simulink model "root"  (R2014a)
settings: Solver=FixedStepDiscrete  StartTime=0.0  StopTime=1  RelTol=1e-3
model workspace (MAT data in the model file):
  Fs = 48000
  dtmfFramesize = 256
undefined symbols (not defined in the file): jet
libraries: DSPBAPrim x6, dspsnks4 x2, dspspect3 x1, dspmathops x1, dspswit3 x1
settings Model: Creator=User  LastModifiedBy=User
settings OptimizationCC: BlockReduction=off  ConditionallyExecuteInputs=off  InlineParams=on
settings HardwareCC: ProdHWDeviceType=ASIC/FPGA->ASIC/FPGA  TargetLongLongMode=on  TargetIntDivRoundTo=Zero  TargetEndianess=LittleEndian  TargetHWDeviceType=MATLAB Host  ProdEqTarget=off

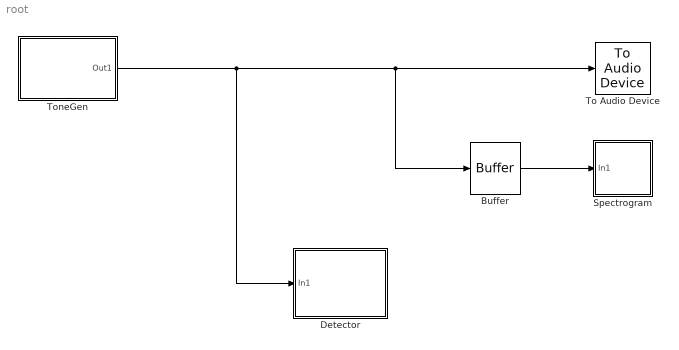
== system root ==
  Buffer : Buffer  N=dtmfFramesize  TreatMby1Signals=One channel
  Detector : Subsystem
  Spectrogram : Subsystem
  To Audio Device : dspsnks4/To Audio Device  deviceName=Default  inheritSampleRate=on  sampleRate=44100  deviceDatatype=Determine from input data type  autoBufferSize=on  bufferSize=4096  queueDuration=1.0  defaultOutputChannelMapping=on  outputChannelMapping=1
  ToneGen : Subsystem
  wires:
  ToneGen/1(Out1) -> Detector/1(In1), Buffer/1, To Audio Device/1
  Buffer/1 -> Spectrogram/1(In1)

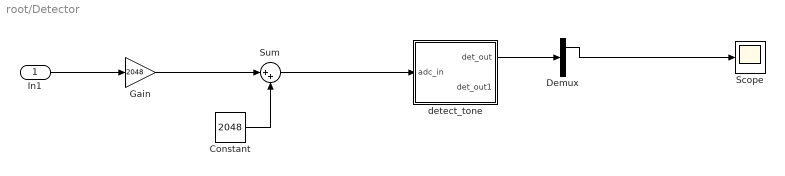
== system root/Detector ==
  In1 : Inport
  Constant : Constant  Value=2048  OutDataTypeStr=fixdt(0,12,0)
  Demux : Demux  Outputs=3
  Gain : Gain  Gain=2048
  Scope : Scope
      settings: YMin=1  YMax=1  MaxDataPoints=500000
  Sum : Sum  Inputs=|++  OutDataTypeStr=fixdt(0,12,0)
  detect_tone : Subsystem
  wires:
  In1/1 -> Gain/1
  Gain/1 -> Sum/1
  Constant/1 -> Sum/2
  Sum/1 -> detect_tone/1(adc_in)
  detect_tone/1(det_out) -> Demux/1
  Demux/1 -> Scope/1

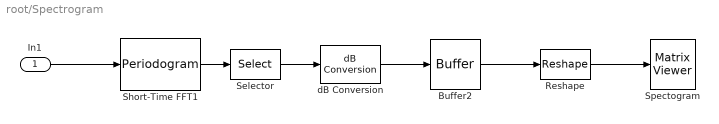
== system root/Spectrogram ==
  In1 : Inport
  Buffer2 : Buffer  N=48*64  V=46*64  ic=-70  TreatMby1Signals=One channel
  Reshape : Reshape  OutputDimensionality=Customize  OutputDimensions=[64 48]
  Selector : Selector  InputPortWidth=dtmfFramesize/2  Indices=1:(dtmfFramesize/4)
  Short-Time FFT1 : dspspect3/Periodogram  measurement=Power spectral density  wintype=Hamming  Rs=50  beta=5  winsamp=Periodic  FFTImplementation=Auto  inheritFFT=off  fftsize=128  navg=2  inheritTs=on  Ts=1
  Spectogram : dspsnks4/Matrix Viewer  ImageParams=on  CMapStr=jet(256)  AxisColorbar=off  AxisParams=on  AxisOrigin=Lower left corner  XLabel=Time Index  YLabel=Frequency Index  ZLabel=dB Magnitude  FigPos=[214 452 283 114]  AxisZoom=on
      settings: YMin=-150  YMax=-65
  dB Conversion : dspmathops/dB Conversion  dBtype=dB  intype=Amplitude  R=1  fuzz=on
  wires:
  Short-Time FFT1/1 -> Selector/1
  Selector/1 -> dB Conversion/1
  Buffer2/1 -> Reshape/1
  In1/1 -> Short-Time FFT1/1
  Reshape/1 -> Spectogram/1
  dB Conversion/1 -> Buffer2/1

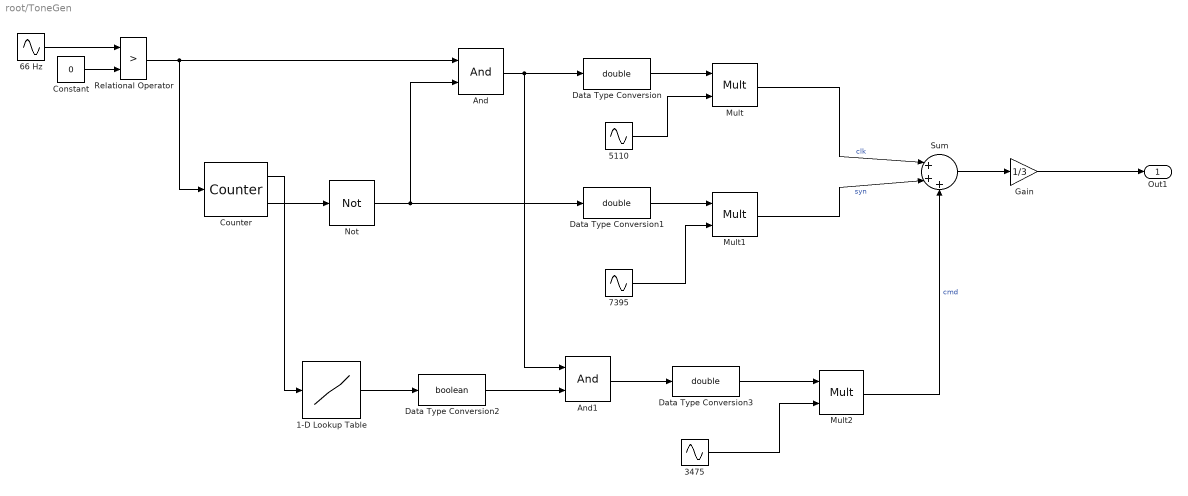
== system root/ToneGen ==
  1-D Lookup Table : Lookup_n-D  NumberOfTableDimensions=1  BreakpointsForDimension1=[0:15]  Table=[0 1 0 1 1 0 1 0 0 1 0 1 0 0 1 1]  InternalRulePriority=Speed  RndMeth=Simplest  InputSameDT=on
  3475 : Sin  Frequency=3475*2*pi  SampleTime=1/Fs
  5110 : Sin  Frequency=5110*2*pi  SampleTime=1/Fs
  66 Hz : Sin  Frequency=66*2*pi  SampleTime=1/Fs
  7395 : Sin  Frequency=7395*2*pi  SampleTime=1/Fs
  And : DSPBAPrim/And  primtype=and  nInputs=2  nOutputs=1  omode=Inherit via internal rule  otype=sfix(16)  scale=2^-15  rndmethod=Unbiased  factor=1  satmethod=Symmetric  shift_vec=[0 1 2 -1]  value=0  inPortNames=[' '; ' '; ' '; ' '; ' '; ' '; ' '; ' '; ' '; ' '; ' '; ' '; ' '; ' '; ' '; ' '; ]  outPortNames=[' ']  dspbaimage=dspba_prim.jpg  text=fprintf('&');  style=Optimised  visibilities=8+2  version=20090407
  And1 : DSPBAPrim/And  primtype=and  nInputs=2  nOutputs=1  omode=Inherit via internal rule  otype=sfix(16)  scale=2^-15  rndmethod=Unbiased  factor=1  satmethod=Symmetric  shift_vec=[0 1 2 -1]  value=0  inPortNames=[' '; ' '; ' '; ' '; ' '; ' '; ' '; ' '; ' '; ' '; ' '; ' '; ' '; ' '; ' '; ' '; ]  outPortNames=[' ']  dspbaimage=dspba_prim.jpg  text=fprintf('&');  style=Optimised  visibilities=8+2  version=20090407
  Constant : Constant  Value=0
  Counter : dspswit3/Counter  Direction=Up  CountEvent=Rising edge  CounterSize=User defined  MaxCount=15  InitialCount=0  Output=Count and Hit  HitValue=0  ResetInput=off  SamplesPerFrame=1  Ts=1  CntDtype=double  HitDtype=Logical
  Data Type Conversion : DataTypeConversion  OutDataTypeStr=double
  Data Type Conversion1 : DataTypeConversion  OutDataTypeStr=double
  Data Type Conversion2 : DataTypeConversion  OutDataTypeStr=boolean
  Data Type Conversion3 : DataTypeConversion  OutDataTypeStr=double
  Gain : Gain  Gain=1/3
  Mult : DSPBAPrim/Mult  primtype=mult  nInputs=2  nOutputs=1  omode=Inherit via internal rule  otype=sfix(16)  scale=2^-15  rndmethod=Unbiased  factor=1  satmethod=Symmetric  shift_vec=[0 1 2 -1]  value=0  inPortNames=[' '; ' ';]  outPortNames=[' ']  dspbaimage=dspba_prim.jpg  text=fprintf('X');  style=Optimised  visibilities=8  version=20090407
  Mult1 : DSPBAPrim/Mult  primtype=mult  nInputs=2  nOutputs=1  omode=Inherit via internal rule  otype=sfix(16)  scale=2^-15  rndmethod=Unbiased  factor=1  satmethod=Symmetric  shift_vec=[0 1 2 -1]  value=0  inPortNames=[' '; ' ';]  outPortNames=[' ']  dspbaimage=dspba_prim.jpg  text=fprintf('X');  style=Optimised  visibilities=8  version=20090407
  Mult2 : DSPBAPrim/Mult  primtype=mult  nInputs=2  nOutputs=1  omode=Inherit via internal rule  otype=sfix(16)  scale=2^-15  rndmethod=Unbiased  factor=1  satmethod=Symmetric  shift_vec=[0 1 2 -1]  value=0  inPortNames=[' '; ' ';]  outPortNames=[' ']  dspbaimage=dspba_prim.jpg  text=fprintf('X');  style=Optimised  visibilities=8  version=20090407
  Not : DSPBAPrim/Not  primtype=not  nInputs=1  nOutputs=1  omode=Inherit via internal rule  otype=sfix(16)  scale=2^-15  rndmethod=Unbiased  factor=1  satmethod=Symmetric  shift_vec=[0 1 2 -1]  value=0  inPortNames=[' '; ' ';]  outPortNames=[' ']  dspbaimage=dspba_prim.jpg  text=fprintf('~');  style=Optimised  visibilities=8  version=20090407
  Relational Operator : RelationalOperator  Operator=>  OutDataTypeStr=boolean
  Sum : Sum  Inputs=|+++
  Out1 : Outport
  wires:
  66 Hz/1 -> Relational Operator/1
  Constant/1 -> Relational Operator/2
  Relational Operator/1 -> And/1, Counter/1
  Data Type Conversion/1 -> Mult/1
  5110/1 -> Mult/2
  Counter/2 -> Not/1
  Not/1 -> And/2, Data Type Conversion1/1
  7395/1 -> Mult1/2
  Sum/1 -> Gain/1
  Mult/1 -> Sum/1  "clk"
  Mult1/1 -> Sum/2  "syn"
  Mult2/1 -> Sum/3  "cmd"
  Data Type Conversion1/1 -> Mult1/1
  3475/1 -> Mult2/2
  Counter/1 -> 1-D Lookup Table/1
  1-D Lookup Table/1 -> Data Type Conversion2/1
  And/1 -> And1/1, Data Type Conversion/1
  And1/1 -> Data Type Conversion3/1
  Data Type Conversion2/1 -> And1/2
  Data Type Conversion3/1 -> Mult2/1
  Gain/1 -> Out1/1

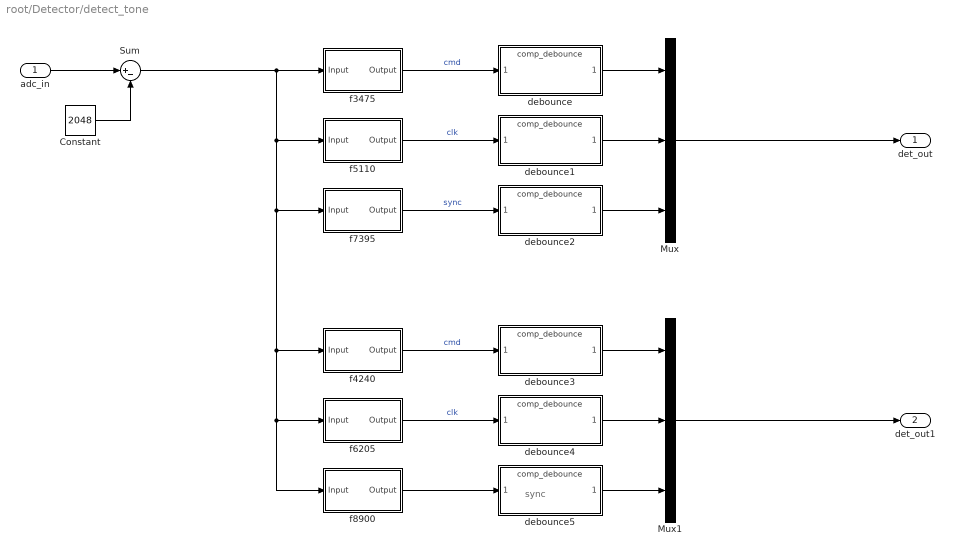
== system root/Detector/detect_tone ==
  note: sync
  adc_in : Inport  OutDataTypeStr=fixdt(0,12,0)
  Constant : Constant  Value=2048  OutDataTypeStr=fixdt(1,16,0)
  Mux : Mux  Inputs=3
  Mux1 : Mux  Inputs=3
  Sum : Sum  Inputs=|+-  AccumDataTypeStr=fixdt(1,16,0)
  debounce{,1..5} (6 alike) : ModelReference  ModelNameDialog=comp_debounce.slx  SimulationMode=Normal  ModelReferenceVersion=1.4  CopyOfModelName=comp_debounce.slx  DefaultDataLogging=on
  f3475 : Subsystem  Tag=FilterWizardSubSystem
      settings: ErrorFcn=dspFilterRealizedInBasicElemsAlgLoopErrFcnCallback
  f4240 : Subsystem  Tag=FilterWizardSubSystem
      settings: ErrorFcn=dspFilterRealizedInBasicElemsAlgLoopErrFcnCallback
  f5110 : Subsystem  Tag=FilterWizardSubSystem
      settings: ErrorFcn=dspFilterRealizedInBasicElemsAlgLoopErrFcnCallback
  f6205 : Subsystem  Tag=FilterWizardSubSystem
      settings: ErrorFcn=dspFilterRealizedInBasicElemsAlgLoopErrFcnCallback
  f7395 : Subsystem  Tag=FilterWizardSubSystem
      settings: ErrorFcn=dspFilterRealizedInBasicElemsAlgLoopErrFcnCallback
  f8900 : Subsystem  Tag=FilterWizardSubSystem
      settings: ErrorFcn=dspFilterRealizedInBasicElemsAlgLoopErrFcnCallback
  det_out : Outport
  det_out1 : Outport  Port=2
  wires:
  adc_in/1 -> Sum/1
  Constant/1 -> Sum/2
  Sum/1 -> f6205/1(Input), f8900/1(Input), f4240/1(Input), f7395/1(Input), f5110/1(Input), f3475/1(Input)
  f3475/1(Output) -> debounce/1  "cmd"
  f5110/1(Output) -> debounce1/1  "clk"
  f7395/1(Output) -> debounce2/1  "sync"
  Mux/1 -> det_out/1
  Mux1/1 -> det_out1/1
  f4240/1(Output) -> debounce3/1  "cmd"
  f6205/1(Output) -> debounce4/1  "clk"
  f8900/1(Output) -> debounce5/1
  debounce/1 -> Mux/1
  debounce1/1 -> Mux/2
  debounce2/1 -> Mux/3
  debounce3/1 -> Mux1/1
  debounce4/1 -> Mux1/2
  debounce5/1 -> Mux1/3

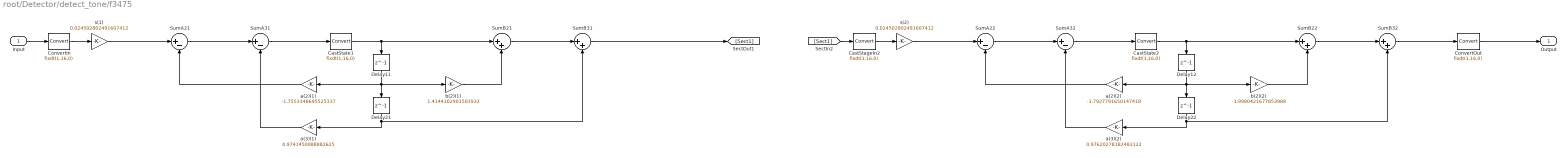
== system root/Detector/detect_tone/f3475 ==
  Input : Inport
  CastStageIn2 : DataTypeConversion  OutDataTypeStr=fixdt(1,16,0)  RndMeth=Convergent  SaturateOnIntegerOverflow=on
  CastState1 : DataTypeConversion  OutDataTypeStr=fixdt(1,16,0)  RndMeth=Convergent  SaturateOnIntegerOverflow=on
  CastState2 : DataTypeConversion  OutDataTypeStr=fixdt(1,16,0)  RndMeth=Convergent  SaturateOnIntegerOverflow=on
  ConvertIn : DataTypeConversion  OutDataTypeStr=fixdt(1,16,0)  RndMeth=Nearest  SaturateOnIntegerOverflow=on
  ConvertOut : DataTypeConversion  OutDataTypeStr=fixdt(1,16,0)  RndMeth=Convergent  SaturateOnIntegerOverflow=on
  Delay{11..12,21..22} (4 alike) : Delay  DelayLength=1  InitialCondition=0
  SumA{21..22,31..32} (4 alike) : Sum  Inputs=|+-  AccumDataTypeStr=fixdt(1,34,14)  OutDataTypeStr=fixdt(1,34,14)  RndMeth=Convergent  SaturateOnIntegerOverflow=on
  SumB{21..22,31..32} (4 alike) : Sum  Inputs=|++  AccumDataTypeStr=fixdt(1,34,14)  OutDataTypeStr=fixdt(1,34,14)  RndMeth=Convergent  SaturateOnIntegerOverflow=on
  a(2)(1) : Gain  Gain=-1.7553348695525337  ParamDataTypeStr=fixdt(1,16,14)  OutDataTypeStr=fixdt(1,32,14)  RndMeth=Convergent  SaturateOnIntegerOverflow=on
  a(2)(2) : Gain  Gain=-1.7927791650147418  ParamDataTypeStr=fixdt(1,16,14)  OutDataTypeStr=fixdt(1,32,14)  RndMeth=Convergent  SaturateOnIntegerOverflow=on
  a(3)(1) : Gain  Gain=0.9741450088882625  ParamDataTypeStr=fixdt(1,16,14)  OutDataTypeStr=fixdt(1,32,14)  RndMeth=Convergent  SaturateOnIntegerOverflow=on
  a(3)(2) : Gain  Gain=0.97620278182483122  ParamDataTypeStr=fixdt(1,16,14)  OutDataTypeStr=fixdt(1,32,14)  RndMeth=Convergent  SaturateOnIntegerOverflow=on
  b(2)(1) : Gain  Gain=1.4144102901503932  ParamDataTypeStr=fixdt(1,16,14)  OutDataTypeStr=fixdt(1,32,14)  RndMeth=Convergent  SaturateOnIntegerOverflow=on
  b(2)(2) : Gain  Gain=-1.9980421677853988  ParamDataTypeStr=fixdt(1,16,14)  OutDataTypeStr=fixdt(1,32,14)  RndMeth=Convergent  SaturateOnIntegerOverflow=on
  s(1) : Gain  Gain=0.024502802491607412  ParamDataTypeStr=fixdt(1,16,20)  OutDataTypeStr=fixdt(1,16,0)  RndMeth=Convergent  SaturateOnIntegerOverflow=on
  s(2) : Gain  Gain=0.024502802491607412  ParamDataTypeStr=fixdt(1,16,20)  OutDataTypeStr=fixdt(1,16,0)  RndMeth=Convergent  SaturateOnIntegerOverflow=on
  Output : Outport
  wires:
  Input/1 -> ConvertIn/1
  s(1)/1 -> SumA21/1
  SumA21/1 -> SumA31/1
  SumA31/1 -> CastState1/1
  CastState1/1 -> SumB21/1, Delay11/1
  SumB21/1 -> SumB31/1
  SumB31/1 -> [Sect1]
  a(2)(1)/1 -> SumA21/2
  Delay11/1 -> a(2)(1)/1, b(2)(1)/1, Delay21/1
  b(2)(1)/1 -> SumB21/2
  a(3)(1)/1 -> SumA31/2
  Delay21/1 -> a(3)(1)/1, SumB31/2
  ConvertIn/1 -> s(1)/1
  [Sect1] -> CastStageIn2/1
  s(2)/1 -> SumA22/1
  SumA22/1 -> SumA32/1
  SumA32/1 -> CastState2/1
  CastState2/1 -> SumB22/1, Delay12/1
  SumB22/1 -> SumB32/1
  SumB32/1 -> ConvertOut/1
  a(2)(2)/1 -> SumA22/2
  Delay12/1 -> a(2)(2)/1, b(2)(2)/1, Delay22/1
  b(2)(2)/1 -> SumB22/2
  a(3)(2)/1 -> SumA32/2
  Delay22/1 -> a(3)(2)/1, SumB32/2
  ConvertOut/1 -> Output/1
  CastStageIn2/1 -> s(2)/1

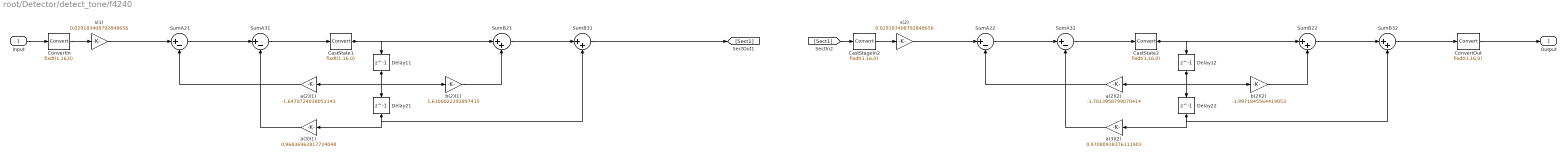
== system root/Detector/detect_tone/f4240 ==
  Input : Inport
  CastStageIn2 : DataTypeConversion  OutDataTypeStr=fixdt(1,16,0)  RndMeth=Convergent  SaturateOnIntegerOverflow=on
  CastState1 : DataTypeConversion  OutDataTypeStr=fixdt(1,16,0)  RndMeth=Convergent  SaturateOnIntegerOverflow=on
  CastState2 : DataTypeConversion  OutDataTypeStr=fixdt(1,16,0)  RndMeth=Convergent  SaturateOnIntegerOverflow=on
  ConvertIn : DataTypeConversion  OutDataTypeStr=fixdt(1,16,0)  RndMeth=Nearest  SaturateOnIntegerOverflow=on
  ConvertOut : DataTypeConversion  OutDataTypeStr=fixdt(1,16,0)  RndMeth=Convergent  SaturateOnIntegerOverflow=on
  Delay{11..12,21..22} (4 alike) : Delay  DelayLength=1  InitialCondition=0
  SumA{21..22,31..32} (4 alike) : Sum  Inputs=|+-  AccumDataTypeStr=fixdt(1,34,14)  OutDataTypeStr=fixdt(1,34,14)  RndMeth=Convergent  SaturateOnIntegerOverflow=on
  SumB{21..22,31..32} (4 alike) : Sum  Inputs=|++  AccumDataTypeStr=fixdt(1,34,14)  OutDataTypeStr=fixdt(1,34,14)  RndMeth=Convergent  SaturateOnIntegerOverflow=on
  a(2)(1) : Gain  Gain=-1.6470724038051143  ParamDataTypeStr=fixdt(1,16,14)  OutDataTypeStr=fixdt(1,32,14)  RndMeth=Convergent  SaturateOnIntegerOverflow=on
  a(2)(2) : Gain  Gain=-1.7013958799070414  ParamDataTypeStr=fixdt(1,16,14)  OutDataTypeStr=fixdt(1,32,14)  RndMeth=Convergent  SaturateOnIntegerOverflow=on
  a(3)(1) : Gain  Gain=0.96836962817724048  ParamDataTypeStr=fixdt(1,16,14)  OutDataTypeStr=fixdt(1,32,14)  RndMeth=Convergent  SaturateOnIntegerOverflow=on
  a(3)(2) : Gain  Gain=0.97080938376111903  ParamDataTypeStr=fixdt(1,16,14)  OutDataTypeStr=fixdt(1,32,14)  RndMeth=Convergent  SaturateOnIntegerOverflow=on
  b(2)(1) : Gain  Gain=1.6100022392897415  ParamDataTypeStr=fixdt(1,16,14)  OutDataTypeStr=fixdt(1,32,14)  RndMeth=Convergent  SaturateOnIntegerOverflow=on
  b(2)(2) : Gain  Gain=-1.9971845564419053  ParamDataTypeStr=fixdt(1,16,14)  OutDataTypeStr=fixdt(1,32,14)  RndMeth=Convergent  SaturateOnIntegerOverflow=on
  s(1) : Gain  Gain=0.029183408792848656  ParamDataTypeStr=fixdt(1,16,20)  OutDataTypeStr=fixdt(1,16,0)  RndMeth=Convergent  SaturateOnIntegerOverflow=on
  s(2) : Gain  Gain=0.029183408792848656  ParamDataTypeStr=fixdt(1,16,20)  OutDataTypeStr=fixdt(1,16,0)  RndMeth=Convergent  SaturateOnIntegerOverflow=on
  Output : Outport
  wires:
  Input/1 -> ConvertIn/1
  s(1)/1 -> SumA21/1
  SumA21/1 -> SumA31/1
  SumA31/1 -> CastState1/1
  CastState1/1 -> SumB21/1, Delay11/1
  SumB21/1 -> SumB31/1
  SumB31/1 -> [Sect1]
  a(2)(1)/1 -> SumA21/2
  Delay11/1 -> a(2)(1)/1, b(2)(1)/1, Delay21/1
  b(2)(1)/1 -> SumB21/2
  a(3)(1)/1 -> SumA31/2
  Delay21/1 -> a(3)(1)/1, SumB31/2
  ConvertIn/1 -> s(1)/1
  [Sect1] -> CastStageIn2/1
  s(2)/1 -> SumA22/1
  SumA22/1 -> SumA32/1
  SumA32/1 -> CastState2/1
  CastState2/1 -> SumB22/1, Delay12/1
  SumB22/1 -> SumB32/1
  SumB32/1 -> ConvertOut/1
  a(2)(2)/1 -> SumA22/2
  Delay12/1 -> a(2)(2)/1, b(2)(2)/1, Delay22/1
  b(2)(2)/1 -> SumB22/2
  a(3)(2)/1 -> SumA32/2
  Delay22/1 -> a(3)(2)/1, SumB32/2
  ConvertOut/1 -> Output/1
  CastStageIn2/1 -> s(2)/1

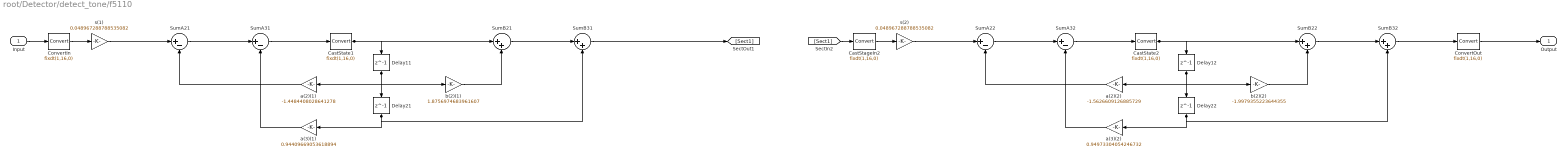
== system root/Detector/detect_tone/f5110 ==
  Input : Inport
  CastStageIn2 : DataTypeConversion  OutDataTypeStr=fixdt(1,16,0)  RndMeth=Convergent  SaturateOnIntegerOverflow=on
  CastState1 : DataTypeConversion  OutDataTypeStr=fixdt(1,16,0)  RndMeth=Convergent  SaturateOnIntegerOverflow=on
  CastState2 : DataTypeConversion  OutDataTypeStr=fixdt(1,16,0)  RndMeth=Convergent  SaturateOnIntegerOverflow=on
  ConvertIn : DataTypeConversion  OutDataTypeStr=fixdt(1,16,0)  RndMeth=Nearest  SaturateOnIntegerOverflow=on
  ConvertOut : DataTypeConversion  OutDataTypeStr=fixdt(1,16,0)  RndMeth=Convergent  SaturateOnIntegerOverflow=on
  Delay{11..12,21..22} (4 alike) : Delay  DelayLength=1  InitialCondition=0
  SumA{21..22,31..32} (4 alike) : Sum  Inputs=|+-  AccumDataTypeStr=fixdt(1,34,14)  OutDataTypeStr=fixdt(1,34,14)  RndMeth=Convergent  SaturateOnIntegerOverflow=on
  SumB{21..22,31..32} (4 alike) : Sum  Inputs=|++  AccumDataTypeStr=fixdt(1,34,14)  OutDataTypeStr=fixdt(1,34,14)  RndMeth=Convergent  SaturateOnIntegerOverflow=on
  a(2)(1) : Gain  Gain=-1.4484408028641278  ParamDataTypeStr=fixdt(1,16,14)  OutDataTypeStr=fixdt(1,32,14)  RndMeth=Convergent  SaturateOnIntegerOverflow=on
  a(2)(2) : Gain  Gain=-1.5626609126885729  ParamDataTypeStr=fixdt(1,16,14)  OutDataTypeStr=fixdt(1,32,14)  RndMeth=Convergent  SaturateOnIntegerOverflow=on
  a(3)(1) : Gain  Gain=0.94409669053618894  ParamDataTypeStr=fixdt(1,16,14)  OutDataTypeStr=fixdt(1,32,14)  RndMeth=Convergent  SaturateOnIntegerOverflow=on
  a(3)(2) : Gain  Gain=0.94973304054246732  ParamDataTypeStr=fixdt(1,16,14)  OutDataTypeStr=fixdt(1,32,14)  RndMeth=Convergent  SaturateOnIntegerOverflow=on
  b(2)(1) : Gain  Gain=1.8756974683961607  ParamDataTypeStr=fixdt(1,16,14)  OutDataTypeStr=fixdt(1,32,14)  RndMeth=Convergent  SaturateOnIntegerOverflow=on
  b(2)(2) : Gain  Gain=-1.9979355223644355  ParamDataTypeStr=fixdt(1,16,14)  OutDataTypeStr=fixdt(1,32,14)  RndMeth=Convergent  SaturateOnIntegerOverflow=on
  s(1) : Gain  Gain=0.048967288788535082  ParamDataTypeStr=fixdt(1,16,19)  OutDataTypeStr=fixdt(1,16,0)  RndMeth=Convergent  SaturateOnIntegerOverflow=on
  s(2) : Gain  Gain=0.048967288788535082  ParamDataTypeStr=fixdt(1,16,19)  OutDataTypeStr=fixdt(1,16,0)  RndMeth=Convergent  SaturateOnIntegerOverflow=on
  Output : Outport
  wires:
  Input/1 -> ConvertIn/1
  s(1)/1 -> SumA21/1
  SumA21/1 -> SumA31/1
  SumA31/1 -> CastState1/1
  CastState1/1 -> SumB21/1, Delay11/1
  SumB21/1 -> SumB31/1
  SumB31/1 -> [Sect1]
  a(2)(1)/1 -> SumA21/2
  Delay11/1 -> a(2)(1)/1, b(2)(1)/1, Delay21/1
  b(2)(1)/1 -> SumB21/2
  a(3)(1)/1 -> SumA31/2
  Delay21/1 -> a(3)(1)/1, SumB31/2
  ConvertIn/1 -> s(1)/1
  [Sect1] -> CastStageIn2/1
  s(2)/1 -> SumA22/1
  SumA22/1 -> SumA32/1
  SumA32/1 -> CastState2/1
  CastState2/1 -> SumB22/1, Delay12/1
  SumB22/1 -> SumB32/1
  SumB32/1 -> ConvertOut/1
  a(2)(2)/1 -> SumA22/2
  Delay12/1 -> a(2)(2)/1, b(2)(2)/1, Delay22/1
  b(2)(2)/1 -> SumB22/2
  a(3)(2)/1 -> SumA32/2
  Delay22/1 -> a(3)(2)/1, SumB32/2
  ConvertOut/1 -> Output/1
  CastStageIn2/1 -> s(2)/1

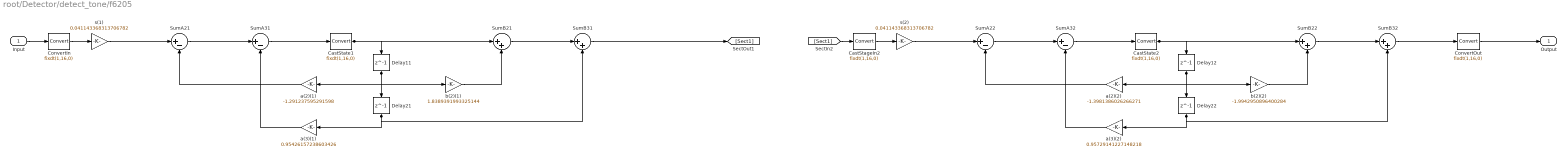
== system root/Detector/detect_tone/f6205 ==
  Input : Inport
  CastStageIn2 : DataTypeConversion  OutDataTypeStr=fixdt(1,16,0)  RndMeth=Convergent  SaturateOnIntegerOverflow=on
  CastState1 : DataTypeConversion  OutDataTypeStr=fixdt(1,16,0)  RndMeth=Convergent  SaturateOnIntegerOverflow=on
  CastState2 : DataTypeConversion  OutDataTypeStr=fixdt(1,16,0)  RndMeth=Convergent  SaturateOnIntegerOverflow=on
  ConvertIn : DataTypeConversion  OutDataTypeStr=fixdt(1,16,0)  RndMeth=Nearest  SaturateOnIntegerOverflow=on
  ConvertOut : DataTypeConversion  OutDataTypeStr=fixdt(1,16,0)  RndMeth=Convergent  SaturateOnIntegerOverflow=on
  Delay{11..12,21..22} (4 alike) : Delay  DelayLength=1  InitialCondition=0
  SumA{21..22,31..32} (4 alike) : Sum  Inputs=|+-  AccumDataTypeStr=fixdt(1,34,14)  OutDataTypeStr=fixdt(1,34,14)  RndMeth=Convergent  SaturateOnIntegerOverflow=on
  SumB{21..22,31..32} (4 alike) : Sum  Inputs=|++  AccumDataTypeStr=fixdt(1,34,14)  OutDataTypeStr=fixdt(1,34,14)  RndMeth=Convergent  SaturateOnIntegerOverflow=on
  a(2)(1) : Gain  Gain=-1.291237595291598  ParamDataTypeStr=fixdt(1,16,14)  OutDataTypeStr=fixdt(1,32,14)  RndMeth=Convergent  SaturateOnIntegerOverflow=on
  a(2)(2) : Gain  Gain=-1.3981386026266271  ParamDataTypeStr=fixdt(1,16,14)  OutDataTypeStr=fixdt(1,32,14)  RndMeth=Convergent  SaturateOnIntegerOverflow=on
  a(3)(1) : Gain  Gain=0.95426157238603426  ParamDataTypeStr=fixdt(1,16,14)  OutDataTypeStr=fixdt(1,32,14)  RndMeth=Convergent  SaturateOnIntegerOverflow=on
  a(3)(2) : Gain  Gain=0.95729141227148218  ParamDataTypeStr=fixdt(1,16,14)  OutDataTypeStr=fixdt(1,32,14)  RndMeth=Convergent  SaturateOnIntegerOverflow=on
  b(2)(1) : Gain  Gain=1.8389391993325144  ParamDataTypeStr=fixdt(1,16,14)  OutDataTypeStr=fixdt(1,32,14)  RndMeth=Convergent  SaturateOnIntegerOverflow=on
  b(2)(2) : Gain  Gain=-1.9942950896400284  ParamDataTypeStr=fixdt(1,16,14)  OutDataTypeStr=fixdt(1,32,14)  RndMeth=Convergent  SaturateOnIntegerOverflow=on
  s(1) : Gain  Gain=0.041143368313706782  ParamDataTypeStr=fixdt(1,16,19)  OutDataTypeStr=fixdt(1,16,0)  RndMeth=Convergent  SaturateOnIntegerOverflow=on
  s(2) : Gain  Gain=0.041143368313706782  ParamDataTypeStr=fixdt(1,16,19)  OutDataTypeStr=fixdt(1,16,0)  RndMeth=Convergent  SaturateOnIntegerOverflow=on
  Output : Outport
  wires:
  Input/1 -> ConvertIn/1
  s(1)/1 -> SumA21/1
  SumA21/1 -> SumA31/1
  SumA31/1 -> CastState1/1
  CastState1/1 -> SumB21/1, Delay11/1
  SumB21/1 -> SumB31/1
  SumB31/1 -> [Sect1]
  a(2)(1)/1 -> SumA21/2
  Delay11/1 -> a(2)(1)/1, b(2)(1)/1, Delay21/1
  b(2)(1)/1 -> SumB21/2
  a(3)(1)/1 -> SumA31/2
  Delay21/1 -> a(3)(1)/1, SumB31/2
  ConvertIn/1 -> s(1)/1
  [Sect1] -> CastStageIn2/1
  s(2)/1 -> SumA22/1
  SumA22/1 -> SumA32/1
  SumA32/1 -> CastState2/1
  CastState2/1 -> SumB22/1, Delay12/1
  SumB22/1 -> SumB32/1
  SumB32/1 -> ConvertOut/1
  a(2)(2)/1 -> SumA22/2
  Delay12/1 -> a(2)(2)/1, b(2)(2)/1, Delay22/1
  b(2)(2)/1 -> SumB22/2
  a(3)(2)/1 -> SumA32/2
  Delay22/1 -> a(3)(2)/1, SumB32/2
  ConvertOut/1 -> Output/1
  CastStageIn2/1 -> s(2)/1

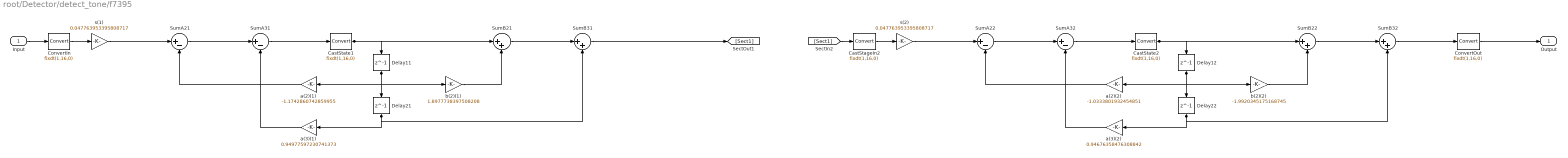
== system root/Detector/detect_tone/f7395 ==
  Input : Inport
  CastStageIn2 : DataTypeConversion  OutDataTypeStr=fixdt(1,16,0)  RndMeth=Convergent  SaturateOnIntegerOverflow=on
  CastState1 : DataTypeConversion  OutDataTypeStr=fixdt(1,16,0)  RndMeth=Convergent  SaturateOnIntegerOverflow=on
  CastState2 : DataTypeConversion  OutDataTypeStr=fixdt(1,16,0)  RndMeth=Convergent  SaturateOnIntegerOverflow=on
  ConvertIn : DataTypeConversion  OutDataTypeStr=fixdt(1,16,0)  RndMeth=Nearest  SaturateOnIntegerOverflow=on
  ConvertOut : DataTypeConversion  OutDataTypeStr=fixdt(1,16,0)  RndMeth=Convergent  SaturateOnIntegerOverflow=on
  Delay{11..12,21..22} (4 alike) : Delay  DelayLength=1  InitialCondition=0
  SumA{21..22,31..32} (4 alike) : Sum  Inputs=|+-  AccumDataTypeStr=fixdt(1,34,14)  OutDataTypeStr=fixdt(1,34,14)  RndMeth=Convergent  SaturateOnIntegerOverflow=on
  SumB{21..22,31..32} (4 alike) : Sum  Inputs=|++  AccumDataTypeStr=fixdt(1,34,14)  OutDataTypeStr=fixdt(1,34,14)  RndMeth=Convergent  SaturateOnIntegerOverflow=on
  a(2)(1) : Gain  Gain=-1.1742860742859955  ParamDataTypeStr=fixdt(1,16,14)  OutDataTypeStr=fixdt(1,32,14)  RndMeth=Convergent  SaturateOnIntegerOverflow=on
  a(2)(2) : Gain  Gain=-1.0333801932454851  ParamDataTypeStr=fixdt(1,16,14)  OutDataTypeStr=fixdt(1,32,14)  RndMeth=Convergent  SaturateOnIntegerOverflow=on
  a(3)(1) : Gain  Gain=0.94977597230741373  ParamDataTypeStr=fixdt(1,16,14)  OutDataTypeStr=fixdt(1,32,14)  RndMeth=Convergent  SaturateOnIntegerOverflow=on
  a(3)(2) : Gain  Gain=0.94676358476308842  ParamDataTypeStr=fixdt(1,16,14)  OutDataTypeStr=fixdt(1,32,14)  RndMeth=Convergent  SaturateOnIntegerOverflow=on
  b(2)(1) : Gain  Gain=1.8977738397508208  ParamDataTypeStr=fixdt(1,16,14)  OutDataTypeStr=fixdt(1,32,14)  RndMeth=Convergent  SaturateOnIntegerOverflow=on
  b(2)(2) : Gain  Gain=-1.9920345175168745  ParamDataTypeStr=fixdt(1,16,14)  OutDataTypeStr=fixdt(1,32,14)  RndMeth=Convergent  SaturateOnIntegerOverflow=on
  s(1) : Gain  Gain=0.047763953395808717  ParamDataTypeStr=fixdt(1,16,19)  OutDataTypeStr=fixdt(1,16,0)  RndMeth=Convergent  SaturateOnIntegerOverflow=on
  s(2) : Gain  Gain=0.047763953395808717  ParamDataTypeStr=fixdt(1,16,19)  OutDataTypeStr=fixdt(1,16,0)  RndMeth=Convergent  SaturateOnIntegerOverflow=on
  Output : Outport
  wires:
  Input/1 -> ConvertIn/1
  s(1)/1 -> SumA21/1
  SumA21/1 -> SumA31/1
  SumA31/1 -> CastState1/1
  CastState1/1 -> SumB21/1, Delay11/1
  SumB21/1 -> SumB31/1
  SumB31/1 -> [Sect1]
  a(2)(1)/1 -> SumA21/2
  Delay11/1 -> a(2)(1)/1, b(2)(1)/1, Delay21/1
  b(2)(1)/1 -> SumB21/2
  a(3)(1)/1 -> SumA31/2
  Delay21/1 -> a(3)(1)/1, SumB31/2
  ConvertIn/1 -> s(1)/1
  [Sect1] -> CastStageIn2/1
  s(2)/1 -> SumA22/1
  SumA22/1 -> SumA32/1
  SumA32/1 -> CastState2/1
  CastState2/1 -> SumB22/1, Delay12/1
  SumB22/1 -> SumB32/1
  SumB32/1 -> ConvertOut/1
  a(2)(2)/1 -> SumA22/2
  Delay12/1 -> a(2)(2)/1, b(2)(2)/1, Delay22/1
  b(2)(2)/1 -> SumB22/2
  a(3)(2)/1 -> SumA32/2
  Delay22/1 -> a(3)(2)/1, SumB32/2
  ConvertOut/1 -> Output/1
  CastStageIn2/1 -> s(2)/1

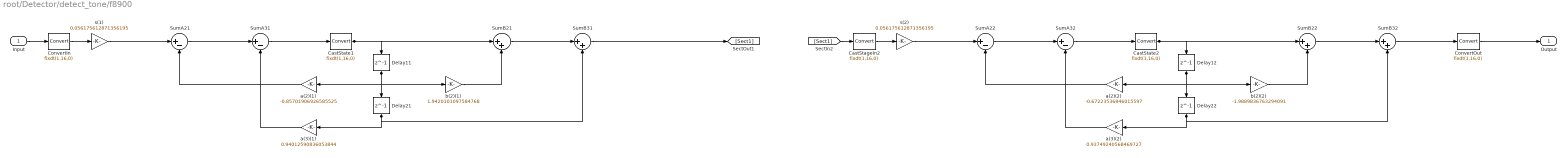
== system root/Detector/detect_tone/f8900 ==
  Input : Inport
  CastStageIn2 : DataTypeConversion  OutDataTypeStr=fixdt(1,16,0)  RndMeth=Convergent  SaturateOnIntegerOverflow=on
  CastState1 : DataTypeConversion  OutDataTypeStr=fixdt(1,16,0)  RndMeth=Convergent  SaturateOnIntegerOverflow=on
  CastState2 : DataTypeConversion  OutDataTypeStr=fixdt(1,16,0)  RndMeth=Convergent  SaturateOnIntegerOverflow=on
  ConvertIn : DataTypeConversion  OutDataTypeStr=fixdt(1,16,0)  RndMeth=Nearest  SaturateOnIntegerOverflow=on
  ConvertOut : DataTypeConversion  OutDataTypeStr=fixdt(1,16,0)  RndMeth=Convergent  SaturateOnIntegerOverflow=on
  Delay{11..12,21..22} (4 alike) : Delay  DelayLength=1  InitialCondition=0
  SumA{21..22,31..32} (4 alike) : Sum  Inputs=|+-  AccumDataTypeStr=fixdt(1,34,14)  OutDataTypeStr=fixdt(1,34,14)  RndMeth=Convergent  SaturateOnIntegerOverflow=on
  SumB{21..22,31..32} (4 alike) : Sum  Inputs=|++  AccumDataTypeStr=fixdt(1,34,14)  OutDataTypeStr=fixdt(1,34,14)  RndMeth=Convergent  SaturateOnIntegerOverflow=on
  a(2)(1) : Gain  Gain=-0.85701906926585525  ParamDataTypeStr=fixdt(1,16,14)  OutDataTypeStr=fixdt(1,32,14)  RndMeth=Convergent  SaturateOnIntegerOverflow=on
  a(2)(2) : Gain  Gain=-0.67223536846015597  ParamDataTypeStr=fixdt(1,16,14)  OutDataTypeStr=fixdt(1,32,14)  RndMeth=Convergent  SaturateOnIntegerOverflow=on
  a(3)(1) : Gain  Gain=0.94012590836053844  ParamDataTypeStr=fixdt(1,16,14)  OutDataTypeStr=fixdt(1,32,14)  RndMeth=Convergent  SaturateOnIntegerOverflow=on
  a(3)(2) : Gain  Gain=0.93749240568469727  ParamDataTypeStr=fixdt(1,16,14)  OutDataTypeStr=fixdt(1,32,14)  RndMeth=Convergent  SaturateOnIntegerOverflow=on
  b(2)(1) : Gain  Gain=1.9420101097584768  ParamDataTypeStr=fixdt(1,16,14)  OutDataTypeStr=fixdt(1,32,14)  RndMeth=Convergent  SaturateOnIntegerOverflow=on
  b(2)(2) : Gain  Gain=-1.9889836763294091  ParamDataTypeStr=fixdt(1,16,14)  OutDataTypeStr=fixdt(1,32,14)  RndMeth=Convergent  SaturateOnIntegerOverflow=on
  s(1) : Gain  Gain=0.056175612871356195  ParamDataTypeStr=fixdt(1,16,19)  OutDataTypeStr=fixdt(1,16,0)  RndMeth=Convergent  SaturateOnIntegerOverflow=on
  s(2) : Gain  Gain=0.056175612871356195  ParamDataTypeStr=fixdt(1,16,19)  OutDataTypeStr=fixdt(1,16,0)  RndMeth=Convergent  SaturateOnIntegerOverflow=on
  Output : Outport
  wires:
  Input/1 -> ConvertIn/1
  s(1)/1 -> SumA21/1
  SumA21/1 -> SumA31/1
  SumA31/1 -> CastState1/1
  CastState1/1 -> SumB21/1, Delay11/1
  SumB21/1 -> SumB31/1
  SumB31/1 -> [Sect1]
  a(2)(1)/1 -> SumA21/2
  Delay11/1 -> a(2)(1)/1, b(2)(1)/1, Delay21/1
  b(2)(1)/1 -> SumB21/2
  a(3)(1)/1 -> SumA31/2
  Delay21/1 -> a(3)(1)/1, SumB31/2
  ConvertIn/1 -> s(1)/1
  [Sect1] -> CastStageIn2/1
  s(2)/1 -> SumA22/1
  SumA22/1 -> SumA32/1
  SumA32/1 -> CastState2/1
  CastState2/1 -> SumB22/1, Delay12/1
  SumB22/1 -> SumB32/1
  SumB32/1 -> ConvertOut/1
  a(2)(2)/1 -> SumA22/2
  Delay12/1 -> a(2)(2)/1, b(2)(2)/1, Delay22/1
  b(2)(2)/1 -> SumB22/2
  a(3)(2)/1 -> SumA32/2
  Delay22/1 -> a(3)(2)/1, SumB32/2
  ConvertOut/1 -> Output/1
  CastStageIn2/1 -> s(2)/1
